simulink model "F16_Model"  (R2023b)
settings: Solver=ode4  StartTime=0.0  StopTime=inf  FixedStep=deltaTime  RelTol=1e-3
PreLoadFcn:
  | addpath(genpath(cd))
InitFcn:
  | Run_Config
undefined symbols (not defined in the file or in its folder): controlDeflections, dataBase, deltaLEF, statesFinal
libraries: simulink_extras x17, vrlib x1, sharedtransform x1
(part 1 of 2)
Description:
  | % Description   :   - Created
  | %                   - Re-arranged blocks.
  | %                   - Added reset in all integrators.
  | %                   - Created Unity Visualizer block.
  | %                   - Created G command to pitch rate
settings Model: SimulationMode=accelerator  Creator=Fatih Erol  LastModifiedBy=cyber
settings DebuggingCC: UnconnectedInputMsg=warning  UnconnectedOutputMsg=warning  UnconnectedLineMsg=warning
settings ModelReferenceCC: EnableRefExpFcnMdlSchedulingChecks=on
settings RTWCC: DLArmComputeVersion=19.05

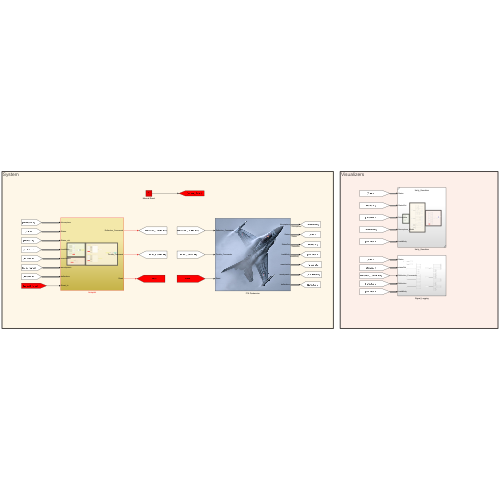
[thumbnail: Simulink's stored preview of the top-level diagram]
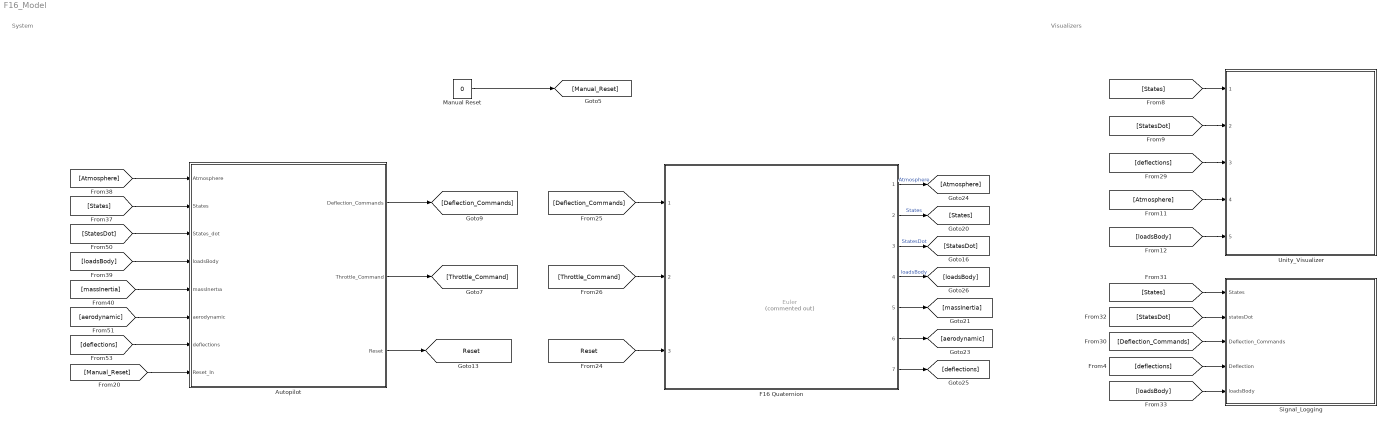
== system F16_Model ==
  note: Visualizers
  note: System
  Autopilot : Subsystem
  Euler : Subsystem  Commented=on
  F16 Quaternion : Subsystem  ReferencedSubsystem=F16_Quaternion
  Manual Reset : Constant  Value=0
      settings: OpenFcn=|
      | val = get_param(gcb,'Value')
      | 
      | switch val
      | case '1'
      | set_param(gcb,'Value','0')
      | set_param(gcb,'BackGroundColor','red')
      | otherwise
      | set_param(gcb,'Value','1')
      | set_param(gcb,'BackGroundColor','green')
      | end
  Signal_Logging : Subsystem
  Unity_Visualizer : Subsystem  ReferencedSubsystem=Unity_Visualizer
  tag scope: Reset=global
  wires:
  [States] -> Unity_Visualizer/1
  [StatesDot] -> Unity_Visualizer/2
  [deflections] -> Unity_Visualizer/3
  [Atmosphere] -> Unity_Visualizer/4
  [loadsBody] -> Unity_Visualizer/5
  [States] -> Signal_Logging/1(States)
  [Deflection_Commands] -> Signal_Logging/3(Deflection_Commands)
  [deflections] -> Signal_Logging/4(Deflection)
  [StatesDot] -> Signal_Logging/2(statesDot)
  [loadsBody] -> Signal_Logging/5(loadsBody)
  [Reset] -> F16 Quaternion/3
  [Throttle_Command] -> F16 Quaternion/2
  [Deflection_Commands] -> F16 Quaternion/1
  F16 Quaternion/7 -> [deflections]
  F16 Quaternion/6 -> [aerodynamic]
  F16 Quaternion/5 -> [massInertia]
  F16 Quaternion/4 -> [loadsBody]  "loadsBody"
  F16 Quaternion/1 -> [Atmosphere]  "Atmosphere"
  F16 Quaternion/3 -> [StatesDot]  "StatesDot"
  F16 Quaternion/2 -> [States]  "States"
  [Atmosphere] -> Autopilot/1(Atmosphere)
  [States] -> Autopilot/2(States)
  [StatesDot] -> Autopilot/3(States_dot)
  [loadsBody] -> Autopilot/4(loadsBody)
  [massInertia] -> Autopilot/5(massInertıa)
  [aerodynamic] -> Autopilot/6(aerodynamic)
  [deflections] -> Autopilot/7(deflections)
  Autopilot/2(Throttle_Command) -> [Throttle_Command]
  Autopilot/1(Deflection_Commands) -> [Deflection_Commands]
  [Manual_Reset] -> Autopilot/8(Reset_In)
  Manual Reset/1 -> [Manual_Reset]
  Autopilot/3(Reset) -> [Reset]

== system F16_Model/Autopilot ==
  note: Outputs
  note: Inputs
  note: Controllers
  Atmosphere : Inport
  States : Inport  Port=2
  States_dot : Inport  Port=3
  loadsBody : Inport  Port=4
  massInertıa : Inport  Port=5
  aerodynamic : Inport  Port=6
  deflections : Inport  Port=7
  Reset_In : Inport  Port=8
  Bus Selector : BusSelector  OutputSignals=deflectionCommands,throttleCommand
  Constant : Constant
  Controller Selector : If  IfExpression=u1 == 1  ElseIfExpressions=u1 == 2  ShowElse=off
  From19 : From  Commented=on  GotoTag=Joystick_Commands
  Joystick : Subsystem  Commented=on
  Merge : Merge
  Simulink Inputs : Subsystem
  Deflection_Commands : Outport
  Throttle_Command : Outport  Port=2
  Reset : Outport  Port=3
  wires:
  aerodynamic/1 -> [aerodynamic]
  loadsBody/1 -> [loadsBody]
  Atmosphere/1 -> [Atmosphere]
  States_dot/1 -> [StatesDot]
  deflections/1 -> [deflections]
  massInertıa/1 -> [massInertia]
  States/1 -> [States]
  [States] -> Simulink Inputs/1(States)
  [Atmosphere] -> Simulink Inputs/3(Atmosphere)
  [loadsBody] -> Simulink Inputs/4(loadsBody)
  [StatesDot] -> Simulink Inputs/2(States_dot)
  [aerodynamic] -> Simulink Inputs/5(aerodynamic)
  [massInertia] -> Simulink Inputs/6(massInertia)
  Reset_In/1 -> [Reset]
  [Reset] -> Simulink Inputs/7(Reset)
  [deflections] -> Simulink Inputs/8(deflections)
  [Manual_Controller_Commands] -> Merge/1
  [Commands] -> Bus Selector/1
  Bus Selector/1 -> Deflection_Commands/1  "<deflectionCommands>"
  Bus Selector/2 -> Throttle_Command/1  "<throttleCommand>"
  [deflections] -> Joystick/8(deflections)
  [Reset] -> Joystick/7(Reset)
  [massInertia] -> Joystick/6(massInertia)
  [aerodynamic] -> Joystick/5(aerodynamic)
  [StatesDot] -> Joystick/2(States_dot)
  [loadsBody] -> Joystick/4(loadsBody)
  [Atmosphere] -> Joystick/3(Atmosphere)
  [States] -> Joystick/1(States)
  Controller Selector/2 -> [Joystick_Controller_Active]
  Controller Selector/1 -> [Simulink_Controller_Active]
  Constant/1 -> Controller Selector/1
  [Simulink_Controller_Active] -> Simulink Inputs/Action
  [Joystick_Controller_Active] -> Joystick/Action
  [Reset] -> Reset/1
  Simulink Inputs/1(Commands) -> [Manual_Controller_Commands]
  Joystick/1(Commands) -> [Joystick_Commands]
  From19/1 -> Merge/2
  Merge/1 -> [Commands]

== system F16_Model/Euler ==
  F16 Euler Rotation : Subsystem  Commented=on
      mask Display: image('F16.PNG'); % Use "Edit Image" on toolstrip to change.
  From5 : From  Commented=on  GotoTag=Deflection_Commands
  From7 : From  Commented=on  GotoTag=Throttle_Command
  Goto : Goto  Commented=on  GotoTag=StatesDot
  Goto1 : Goto  Commented=on  GotoTag=States
  Goto11 : Goto  Commented=on  GotoTag=massInertia
  Goto12 : Goto  Commented=on  GotoTag=aerodynamic
  Goto2 : Goto  Commented=on  GotoTag=Atmosphere
  Goto3 : Goto  Commented=on  GotoTag=deflections
  Goto6 : Goto  Commented=on  GotoTag=loadsBody
  Goto8 : Goto  Commented=on  GotoTag=DCMs
  wires:
  F16 Euler Rotation/1(Atmosphere) -> Goto2/1  "Atmosphere"
  F16 Euler Rotation/4(loadsBody) -> Goto6/1  "loadsBody"
  F16 Euler Rotation/6(aerodynamic) -> Goto12/1
  F16 Euler Rotation/7(deflections) -> Goto3/1
  F16 Euler Rotation/3(StatesDot) -> Goto/1  "StatesDot"
  From5/1 -> F16 Euler Rotation/1(Deflection_Commands)
  F16 Euler Rotation/8(DCMs) -> Goto8/1
  F16 Euler Rotation/5(massInertia) -> Goto11/1
  F16 Euler Rotation/2(States) -> Goto1/1  "States"
  From7/1 -> F16 Euler Rotation/2(Throttle_Commands)

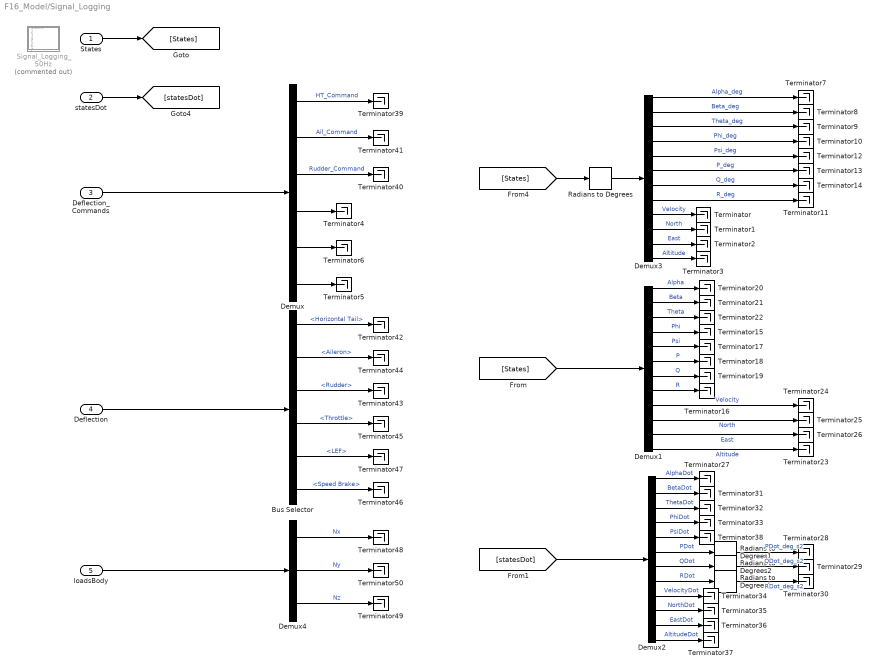
== system F16_Model/Signal_Logging ==
  States : Inport
  statesDot : Inport  Port=2
  Deflection_Commands : Inport  Port=3
  Deflection : Inport  Port=4
  loadsBody : Inport  Port=5
  Bus Selector : BusSelector  OutputSignals=Horizontal Tail,Aileron,Rudder,Throttle,LEF,Speed Brake
  Demux : Demux  Outputs=6
  Demux1 : Demux  Outputs=12
  Demux2 : Demux  Outputs=12
  Demux3 : Demux  Outputs=12
  Demux4 : Demux  Outputs=3
  Radians to Degrees{,1..3} (4 alike) : simulink_extras/Transformations/Radians to Degrees
  Signal_Logging_50Hz : Subsystem  Commented=on
  Terminator{,1..50} (51 alike) : Terminator
  wires:
  Demux3/1 -> Terminator7/1  "Alpha_deg"
  Demux3/5 -> Terminator12/1  "Psi_deg"
  Demux3/10 -> Terminator1/1  "North"
  Demux3/8 -> Terminator11/1  "R_deg"
  Demux3/9 -> Terminator/1  "Velocity"
  Demux3/4 -> Terminator10/1  "Phi_deg"
  [States] -> Radians to Degrees/1
  Demux3/7 -> Terminator14/1  "Q_deg"
  Demux3/11 -> Terminator2/1  "East"
  Demux3/6 -> Terminator13/1  "P_deg"
  Demux3/3 -> Terminator9/1  "Theta_deg"
  Radians to Degrees/1 -> Demux3/1
  Demux3/2 -> Terminator8/1  "Beta_deg"
  Demux3/12 -> Terminator3/1  "Altitude"
  States/1 -> [States]
  Deflection_Commands/1 -> Demux/1
  Demux/5 -> Terminator6/1
  Demux/2 -> Terminator41/1  "Ail_Command"
  Demux/1 -> Terminator39/1  "HT_Command"
  Demux/6 -> Terminator5/1
  Demux/4 -> Terminator4/1
  Demux/3 -> Terminator40/1  "Rudder_Command"
  [States] -> Demux1/1
  Demux1/2 -> Terminator21/1  "Beta"
  Demux1/3 -> Terminator22/1  "Theta"
  Demux1/6 -> Terminator18/1  "P"
  Demux1/7 -> Terminator19/1  "Q"
  Demux1/4 -> Terminator15/1  "Phi"
  Demux1/8 -> Terminator16/1  "R"
  Demux1/5 -> Terminator17/1  "Psi"
  Demux1/1 -> Terminator20/1  "Alpha"
  Demux1/9 -> Terminator24/1  "Velocity"
  Demux1/10 -> Terminator25/1  "North"
  Demux1/11 -> Terminator26/1  "East"
  Demux1/12 -> Terminator23/1  "Altitude"
  statesDot/1 -> [statesDot]
  Demux2/8 -> Radians to Degrees3/1  "RDot"
  Demux4/3 -> Terminator49/1  "Nz"
  [statesDot] -> Demux2/1
  Demux2/9 -> Terminator34/1  "VelocityDot"
  Demux4/2 -> Terminator50/1  "Ny"
  Demux4/1 -> Terminator48/1  "Nx"
  Demux2/5 -> Terminator38/1  "PsiDot"
  Demux2/11 -> Terminator36/1  "EastDot"
  Demux2/6 -> Radians to Degrees1/1  "PDot"
  Demux2/7 -> Radians to Degrees2/1  "QDot"
  Demux2/10 -> Terminator35/1  "NorthDot"
  Demux2/4 -> Terminator33/1  "PhiDot"
  Demux2/2 -> Terminator31/1  "BetaDot"
  Demux2/3 -> Terminator32/1  "ThetaDot"
  Demux2/1 -> Terminator27/1  "AlphaDot"
  loadsBody/1 -> Demux4/1
  Demux2/12 -> Terminator37/1  "AltitudeDot"
  Radians to Degrees1/1 -> Terminator28/1  "PDot_deg_s2"
  Radians to Degrees2/1 -> Terminator29/1  "QDot_deg_s2"
  Radians to Degrees3/1 -> Terminator30/1  "RDot_deg_s2"
  Deflection/1 -> Bus Selector/1
  Bus Selector/1 -> Terminator42/1  "<Horizontal Tail>"
  Bus Selector/2 -> Terminator44/1  "<Aileron>"
  Bus Selector/3 -> Terminator43/1  "<Rudder>"
  Bus Selector/4 -> Terminator45/1  "<Throttle>"
  Bus Selector/5 -> Terminator47/1  "<LEF>"
  Bus Selector/6 -> Terminator46/1  "<Speed Brake>"

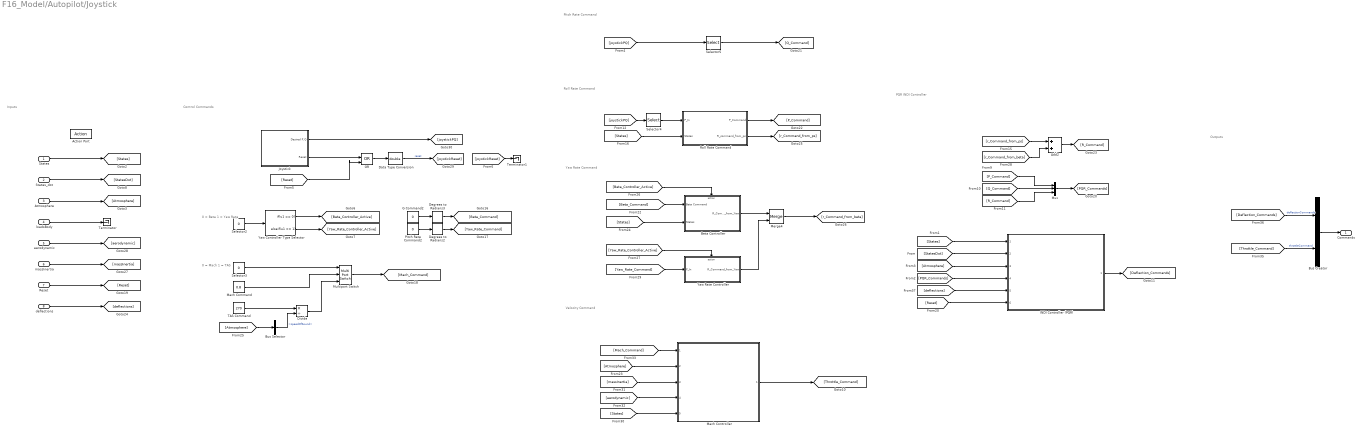
== system F16_Model/Autopilot/Joystick ==
  note: PQR INDI Controller
  note: Velocity Command
  note: Yaw Rate Command
  note: Roll Rate Command
  note: 0 = Mach
      | 1 = TAS
  note: Inputs
  note: Outputs
  note: Control Commands
  note: 0 = Beta
      | 1 = Yaw Rate
  note: Pitch Rate Command
  States : Inport
  States_dot : Inport  Port=2
  Atmosphere : Inport  Port=3
  loadsBody : Inport  Port=4
  aerodynamic : Inport  Port=5
  massInertia : Inport  Port=6
  Reset : Inport  Port=7
  deflections : Inport  Port=8
  Action Port : ActionPort  ActionPortLabel=elseif(u1 == 2)
  Add2 : Sum
  Beta Controller : Subsystem  TreatAsAtomicUnit=on
  Bus Creator : BusCreator  Inputs=2
  Bus Selector : BusSelector  OutputSignals=speedOfSound
  Data Type Conversion : DataTypeConversion  OutDataTypeStr=double  SaturateOnIntegerOverflow=off  RndMeth=Floor
  Degrees to Radians2 : simulink_extras/Transformations/Degrees to Radians
  Degrees to Radians3 : simulink_extras/Transformations/Degrees to Radians
  Divide : Product  Inputs=*/
  G Command2 : Constant  Value=0
  INDI Controller (PQR) : Subsystem  ReferencedSubsystem=INDI_Controller_PQR
  Joystick : Subsystem
  Mach Command : Constant  Value=0.8
  Mach Controller : Subsystem  ReferencedSubsystem=Mach_Controller
  Merge4 : Merge
  Multiport Switch : MultiPortSwitch  DataPortOrder=Zero-based contiguous  Inputs=2  zeroidx=on  SaturateOnIntegerOverflow=off  InputSameDT=off
  Mux : Mux  Inputs=3
  OR : Logic  Operator=OR  IconShape=distinctive  AllPortsSameDT=off  OutDataTypeStr=boolean
  Pitch Rate Command2 : Constant  Value=0
  Roll Rate Command : Subsystem
  Selector2 : Constant  Value=0
      settings: OpenFcn=|
      | val = get_param(gcb,'Value')
      | 
      | switch val
      | case '1'
      | set_param(gcb,'Value','0')
      | set_param(gcb,'BackGroundColor','red')
      | otherwise
      | set_param(gcb,'Value','1')
      | set_param(gcb,'BackGroundColor','green')
      | end
  Selector3 : Constant  Value=0
      settings: OpenFcn=|
      | val = get_param(gcb,'Value')
      | 
      | switch val
      | case '1'
      | set_param(gcb,'Value','0')
      | set_param(gcb,'BackGroundColor','red')
      | otherwise
      | set_param(gcb,'Value','1')
      | set_param(gcb,'BackGroundColor','green')
      | end
  Selector4 : Selector  InputPortWidth=2  IndexOptions=Index vector (dialog)  Indices=1  OutputSizes=1
  Selector5 : Selector  InputPortWidth=2  IndexOptions=Index vector (dialog)  Indices=2  OutputSizes=1
  TAS Command : Constant  Value=270
  Terminator : Terminator
  Terminator1 : Terminator
  Yaw Controller Type Selector : If  IfExpression=u1 == 0  ElseIfExpressions=u1 == 1  ShowElse=off
  Yaw Rate Controller : Subsystem
  Commands : Outport
  wires:
  Degrees to Radians3/1 -> [Beta_Command]
  deflections/1 -> [deflections]
  Reset/1 -> [Reset]
  INDI Controller (PQR)/1 -> [Deflection_Commands]
  Mach Controller/1 -> [Throttle_Command]
  Mach Command/1 -> Multiport Switch/2
  Divide/1 -> Multiport Switch/3
  Selector3/1 -> Multiport Switch/1
  Multiport Switch/1 -> [Mach_Command]
  TAS Command/1 -> Divide/1
  Bus Selector/1 -> Divide/2  "<speedOfSound>"
  [Atmosphere] -> Bus Selector/1
  aerodynamic/1 -> [aerodynamic]
  massInertia/1 -> [massInertia]
  [aerodynamic] -> Mach Controller/4
  [States] -> Mach Controller/5
  [Mach_Command] -> Mach Controller/1
  [massInertia] -> Mach Controller/3
  [Atmosphere] -> Mach Controller/2
  [Yaw_Rate_Controller_Active] -> Yaw Rate Controller/Action
  [Beta_Controller_Active] -> Beta Controller/Action
  [Yaw_Rate_Command] -> Yaw Rate Controller/1(P_In)
  [Beta_Command] -> Beta Controller/1(Beta Command)
  [States] -> Beta Controller/2(States)
  Beta Controller/1(R_Command_from_Yaw) -> Merge4/1
  Yaw Rate Controller/1(R_Command_from_Yaw) -> Merge4/2
  Merge4/1 -> [r_Command_from_beta]
  [States] -> Roll Rate Command/2(States)
  Add2/1 -> [R_Command]
  [r_Command_from_ps] -> Add2/1
  [r_Command_from_beta] -> Add2/2
  Selector4/1 -> Roll Rate Command/1(P_In)
  Selector5/1 -> [Q_Command]
  [R_Command] -> Mux/3
  [P_Command] -> Mux/1
  [Q_Command] -> Mux/2
  Mux/1 -> [PQR_Commands]
  Degrees to Radians2/1 -> [Yaw_Rate_Command]
  G Command2/1 -> Degrees to Radians3/1
  Pitch Rate Command2/1 -> Degrees to Radians2/1
  Yaw Controller Type Selector/2 -> [Yaw_Rate_Controller_Active]
  Yaw Controller Type Selector/1 -> [Beta_Controller_Active]
  Selector2/1 -> Yaw Controller Type Selector/1
  States_dot/1 -> [StatesDot]
  [Reset] -> INDI Controller (PQR)/6
  [PQR_Commands] -> INDI Controller (PQR)/4
  [deflections] -> INDI Controller (PQR)/5
  [States] -> INDI Controller (PQR)/1
  [StatesDot] -> INDI Controller (PQR)/2
  [Atmosphere] -> INDI Controller (PQR)/3
  States/1 -> [States]
  loadsBody/1 -> Terminator/1
  Atmosphere/1 -> [Atmosphere]
  Joystick/1(Desired P,Q) -> [joystickPQ]
  Joystick/2(Reset) -> OR/1
  [joystickPQ] -> Selector4/1
  Roll Rate Command/2(R_command_from_ps) -> [r_Command_from_ps]
  [joystickPQ] -> Selector5/1
  Roll Rate Command/1(P_Command) -> [P_Command]
  [Deflection_Commands] -> Bus Creator/1  "deflectionCommands"
  [Throttle_Command] -> Bus Creator/2  "throttleCommand"
  Bus Creator/1 -> Commands/1
  [Reset] -> OR/2
  OR/1 -> Data Type Conversion/1
  Data Type Conversion/1 -> [joystickReset]  "reset"
  [joystickReset] -> Terminator1/1

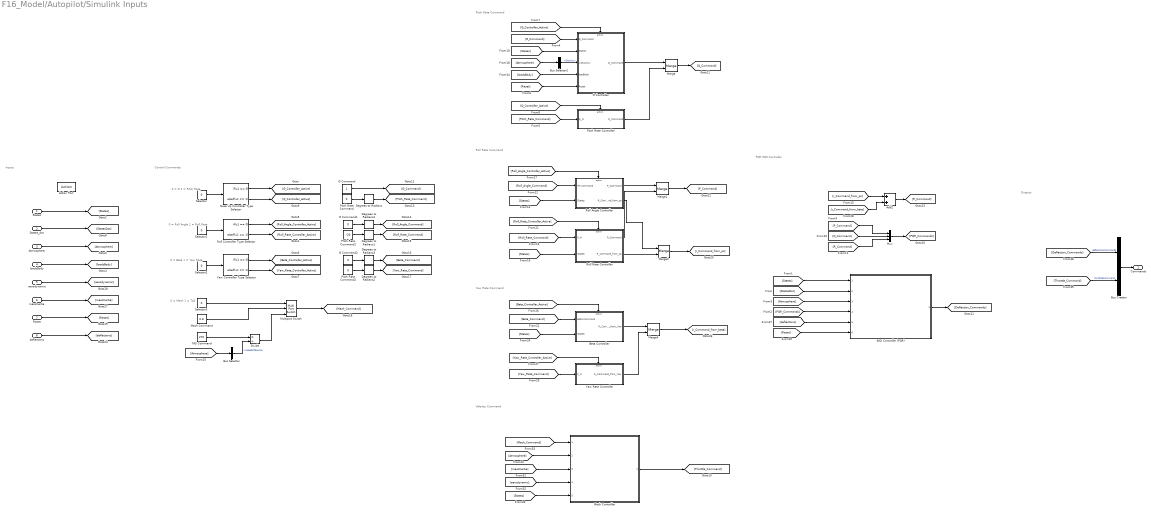
== system F16_Model/Autopilot/Simulink Inputs ==
  note: Pitch Rate Command
  note: 0 = Beta
      | 1 = Yaw Rate
  note: Control Commands
  note: Outputs
  note: Inputs
  note: 0 = G
      | 1 = Pitch Rate
  note: 0 = Roll Angle
      | 1 = Roll Rate
  note: 0 = Mach
      | 1 = TAS
  note: Roll Rate Command
  note: Yaw Rate Command
  note: Velocity Command
  note: PQR INDI Controller
  States : Inport
  States_dot : Inport  Port=2
  Atmosphere : Inport  Port=3
  loadsBody : Inport  Port=4
  aerodynamic : Inport  Port=5
  massInertia : Inport  Port=6
  Reset : Inport  Port=7
  deflections : Inport  Port=8
  Action Port : ActionPort  ActionPortLabel=if(u1 == 1)
  Add2 : Sum
  Beta Controller : Subsystem  TreatAsAtomicUnit=on
  Bus Creator : BusCreator  Inputs=2
  Bus Selector : BusSelector  OutputSignals=speedOfSound
  Bus Selector2 : BusSelector  OutputSignals=Gravity
  Degrees to Radians{,1..4} (5 alike) : simulink_extras/Transformations/Degrees to Radians
  Divide : Product  Inputs=*/
  G Command : Constant
  G Command1 : Constant  Value=0
  G Command2 : Constant  Value=0
  G Controller : Subsystem  TreatAsAtomicUnit=on
  INDI Controller (PQR) : Subsystem  ReferencedSubsystem=INDI_Controller_PQR
  Mach Command : Constant  Value=0.8
  Mach Controller : Subsystem  ReferencedSubsystem=Mach_Controller
  Merge{,1..2,4} (4 alike) : Merge
  Multiport Switch : MultiPortSwitch  DataPortOrder=Zero-based contiguous  Inputs=2  zeroidx=on  SaturateOnIntegerOverflow=off  InputSameDT=off
  Mux : Mux  Inputs=3
  Nose Up Controller Type Selector : If  IfExpression=u1 == 0  ElseIfExpressions=u1 == 1  ShowElse=off
  Pitch Rate Command : Constant  Value=0
  Pitch Rate Command1 : Constant  Value=-20
  Pitch Rate Command2 : Constant  Value=0
  Pitch Rate Controller : Subsystem  TreatAsAtomicUnit=on
  Roll Angle Controller : Subsystem  TreatAsAtomicUnit=on
  Roll Controller Type Selector : If  IfExpression=u1 == 0  ElseIfExpressions=u1 == 1  ShowElse=off
  Roll Rate Controller : Subsystem  TreatAsAtomicUnit=on
  Selector{,1..3} (4 alike) : Constant  Value=0
      settings: OpenFcn=|
      | val = get_param(gcb,'Value')
      | 
      | switch val
      | case '1'
      | set_param(gcb,'Value','0')
      | set_param(gcb,'BackGroundColor','red')
      | otherwise
      | set_param(gcb,'Value','1')
      | set_param(gcb,'BackGroundColor','green')
      | end
  TAS Command : Constant  Value=270
  Yaw Controller Type Selector : If  IfExpression=u1 == 0  ElseIfExpressions=u1 == 1  ShowElse=off
  Yaw Rate Controller : Subsystem
  Commands : Outport
  wires:
  [Atmosphere] -> Bus Selector2/1
  Atmosphere/1 -> [Atmosphere]
  loadsBody/1 -> [loadsBody]
  States/1 -> [States]
  [G_Command] -> G Controller/1(G_Command)
  [States] -> G Controller/2(States)
  Bus Selector2/1 -> G Controller/3(<Gravity>)  "<Gravity>"
  [loadsBody] -> G Controller/4(loadBody)
  [Atmosphere] -> INDI Controller (PQR)/3
  [StatesDot] -> INDI Controller (PQR)/2
  [States] -> INDI Controller (PQR)/1
  [deflections] -> INDI Controller (PQR)/5
  [PQR_Commands] -> INDI Controller (PQR)/4
  [Reset] -> INDI Controller (PQR)/6
  States_dot/1 -> [StatesDot]
  Pitch Rate Command/1 -> Degrees to Radians/1
  Selector1/1 -> Roll Controller Type Selector/1
  Selector2/1 -> Yaw Controller Type Selector/1
  Yaw Controller Type Selector/1 -> [Beta_Controller_Active]
  G Controller/1(Q_Command) -> Merge/1
  Selector/1 -> Nose Up Controller Type Selector/1
  Pitch Rate Controller/1(Q_Command) -> Merge/2
  [Pitch_Rate_Command] -> Pitch Rate Controller/1(Q_In)
  Nose Up Controller Type Selector/1 -> [G_Controller_Active]
  [G_Controller_Active] -> G Controller/Action
  Nose Up Controller Type Selector/2 -> [Q_Controller_Active]
  [Q_Controller_Active] -> Pitch Rate Controller/Action
  Roll Controller Type Selector/1 -> [Roll_Angle_Controller_Active]
  Roll Controller Type Selector/2 -> [Roll_Rate_Controller_Active]
  Yaw Controller Type Selector/2 -> [Yaw_Rate_Controller_Active]
  G Command/1 -> [G_Command]
  Degrees to Radians/1 -> [Pitch_Rate_Command]
  Degrees to Radians1/1 -> [Roll_Rate_Command]
  G Command1/1 -> Degrees to Radians4/1
  Pitch Rate Command1/1 -> Degrees to Radians1/1
  Pitch Rate Command2/1 -> Degrees to Radians2/1
  G Command2/1 -> Degrees to Radians3/1
  Degrees to Radians2/1 -> [Yaw_Rate_Command]
  Mux/1 -> [PQR_Commands]
  [Q_Command] -> Mux/2
  [P_Command] -> Mux/1
  [R_Command] -> Mux/3
  Merge/1 -> [Q_Command]
  Merge1/1 -> [P_Command]
  [Roll_Rate_Controller_Active] -> Roll Rate Controller/Action
  [Roll_Angle_Controller_Active] -> Roll Angle Controller/Action
  [Roll_Rate_Command] -> Roll Rate Controller/1(P_In)
  Roll Rate Controller/1(P_Command) -> Merge1/2
  Roll Angle Controller/1(P_Command) -> Merge1/1
  [Roll_Angle_Command] -> Roll Angle Controller/1(Phi Command)
  [States] -> Roll Angle Controller/2(States)
  [r_Command_from_beta] -> Add2/2
  [r_Command_from_ps] -> Add2/1
  Add2/1 -> [R_Command]
  [States] -> Roll Rate Controller/2(States)
  Roll Angle Controller/2(R_Command_from_ps) -> Merge2/1
  Roll Rate Controller/2(R_command_from_ps) -> Merge2/2
  Merge2/1 -> [r_Command_from_ps]
  Merge4/1 -> [r_Command_from_beta]
  Yaw Rate Controller/1(R_Command_from_Yaw) -> Merge4/2
  Beta Controller/1(R_Command_from_Yaw) -> Merge4/1
  [States] -> Beta Controller/2(States)
  [Beta_Command] -> Beta Controller/1(Beta Command)
  [Yaw_Rate_Command] -> Yaw Rate Controller/1(P_In)
  [Beta_Controller_Active] -> Beta Controller/Action
  [Yaw_Rate_Controller_Active] -> Yaw Rate Controller/Action
  [Atmosphere] -> Mach Controller/2
  [massInertia] -> Mach Controller/3
  [Mach_Command] -> Mach Controller/1
  [States] -> Mach Controller/5
  [aerodynamic] -> Mach Controller/4
  massInertia/1 -> [massInertia]
  aerodynamic/1 -> [aerodynamic]
  [Atmosphere] -> Bus Selector/1
  Bus Selector/1 -> Divide/2  "<speedOfSound>"
  TAS Command/1 -> Divide/1
  Multiport Switch/1 -> [Mach_Command]
  Selector3/1 -> Multiport Switch/1
  Divide/1 -> Multiport Switch/3
  Mach Command/1 -> Multiport Switch/2
  Mach Controller/1 -> [Throttle_Command]
  [Throttle_Command] -> Bus Creator/2  "throttleCommand"
  [Deflection_Commands] -> Bus Creator/1  "deflectionCommands"
  INDI Controller (PQR)/1 -> [Deflection_Commands]
  Reset/1 -> [Reset]
  deflections/1 -> [deflections]
  Degrees to Radians3/1 -> [Beta_Command]
  Degrees to Radians4/1 -> [Roll_Angle_Command]
  Bus Creator/1 -> Commands/1
  [Reset] -> G Controller/5(Reset)

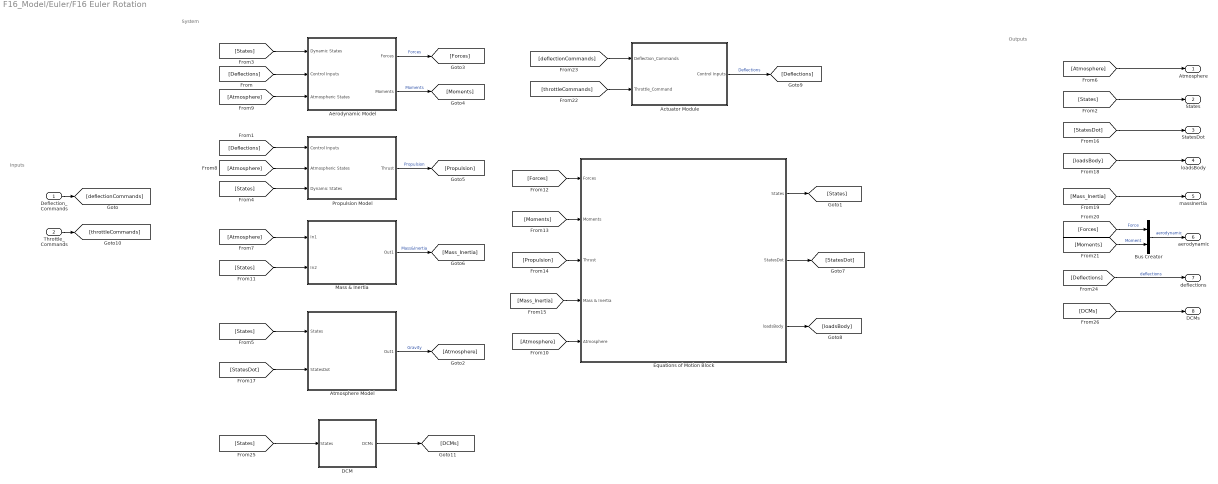
== system F16_Model/Euler/F16 Euler Rotation ==
  note: System
  note: Inputs
  note: Outputs
  Deflection_Commands : Inport
  Throttle_Commands : Inport  Port=2
  Actuator Module : Subsystem
      mask Display: image('F16_ControlSurface.png'); % Use "Edit Image" on toolstrip to change.
  Aerodynamic Model : Subsystem
      mask Display: image('F16.PNG'); % Use "Edit Image" on toolstrip to change.
  Atmosphere Model : Subsystem
      mask Display: image('f16_atm.jpg'); % Use "Edit Image" on toolstrip to change.
  Bus Creator : BusCreator  Inputs=2
  DCM : Subsystem
  Equations of Motion Block : Subsystem
      mask Display: image('F16.PNG'); % Use "Edit Image" on toolstrip to change.
  Mass & Inertia : Subsystem
      mask Display: image('F16.PNG'); % Use "Edit Image" on toolstrip to change.
  Propulsion Model : Subsystem
      mask Display: image('F16_Engine.PNG'); % Use "Edit Image" on toolstrip to change.
  Atmosphere : Outport
  States : Outport  Port=2
  StatesDot : Outport  Port=3
  loadsBody : Outport  Port=4
  massInertia : Outport  Port=5
  aerodynamic : Outport  Port=6
  deflections : Outport  Port=7
  DCMs : Outport  Port=8
  wires:
  Mass & Inertia/1(Out1) -> [Mass_Inertia]  "Mass&Inertia"
  Equations of Motion Block/1(States) -> [States]
  Aerodynamic Model/2(Moments) -> [Moments]  "Moments"
  Aerodynamic Model/1(Forces) -> [Forces]  "Forces"
  [Deflections] -> Aerodynamic Model/2(Control Inputs)
  Atmosphere Model/1(Out1) -> [Atmosphere]  "Gravity"
  Propulsion Model/1(Thrust) -> [Propulsion]  "Propulsion"
  Equations of Motion Block/2(StatesDot) -> [StatesDot]
  Deflection_Commands/1 -> [deflectionCommands]
  [Deflections] -> Propulsion Model/1(Control Inputs)
  [States] -> States/1
  [States] -> Aerodynamic Model/1(Dynamic States)
  [States] -> Propulsion Model/3(Dynamic States)
  [States] -> Atmosphere Model/1(States)
  [Atmosphere] -> Atmosphere/1
  [Atmosphere] -> Mass & Inertia/1(In1)
  [Atmosphere] -> Propulsion Model/2(Atmospheric States)
  [Atmosphere] -> Aerodynamic Model/3(Atmospheric States)
  [Atmosphere] -> Equations of Motion Block/5(Atmosphere)
  [States] -> Mass & Inertia/2(In2)
  [Forces] -> Equations of Motion Block/1(Forces)
  [Moments] -> Equations of Motion Block/2(Moments)
  [Propulsion] -> Equations of Motion Block/3(Thrust)
  [Mass_Inertia] -> Equations of Motion Block/4(Mass & Inertia)
  [StatesDot] -> StatesDot/1
  [StatesDot] -> Atmosphere Model/2(StatesDot)
  Equations of Motion Block/3(loadsBody) -> [loadsBody]
  [loadsBody] -> loadsBody/1
  [Mass_Inertia] -> massInertia/1
  [Forces] -> Bus Creator/1  "Force"
  [Moments] -> Bus Creator/2  "Moment"
  Bus Creator/1 -> aerodynamic/1  "aerodynamic"
  [throttleCommands] -> Actuator Module/2(Throttle_Command)
  Actuator Module/1(Control Inputs) -> [Deflections]  "Deflections"
  [deflectionCommands] -> Actuator Module/1(Deflection_Commands)
  Throttle_Commands/1 -> [throttleCommands]
  [Deflections] -> deflections/1  "deflections"
  [States] -> DCM/1(States)
  DCM/1(DCMs) -> [DCMs]
  [DCMs] -> DCMs/1

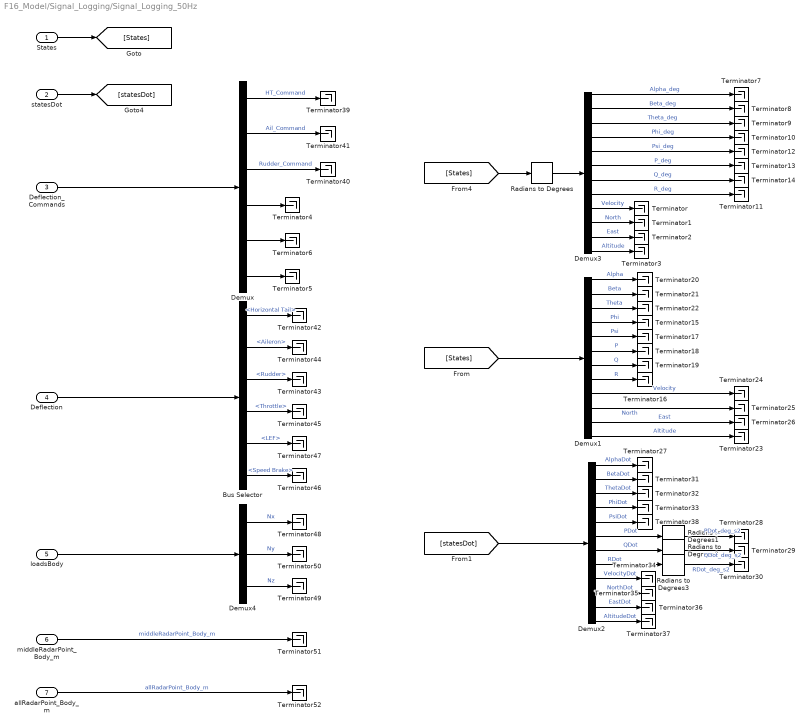
== system F16_Model/Signal_Logging/Signal_Logging_50Hz ==
  States : Inport
  statesDot : Inport  Port=2
  Deflection_Commands : Inport  Port=3
  Deflection : Inport  Port=4
  loadsBody : Inport  Port=5
  middleRadarPoint_Body_m : Inport  Port=6
  allRadarPoint_Body_m : Inport  Port=7
  Bus Selector : BusSelector  OutputSignals=Horizontal Tail,Aileron,Rudder,Throttle,LEF,Speed Brake
  Demux : Demux  Outputs=6
  Demux1 : Demux  Outputs=12
  Demux2 : Demux  Outputs=12
  Demux3 : Demux  Outputs=12
  Demux4 : Demux  Outputs=3
  Radians to Degrees{,1..3} (4 alike) : simulink_extras/Transformations/Radians to Degrees
  Terminator{,1..52} (53 alike) : Terminator
  wires:
  allRadarPoint_Body_m/1 -> Terminator52/1  "allRadarPoint_Body_m"
  middleRadarPoint_Body_m/1 -> Terminator51/1  "middleRadarPoint_Body_m"
  Bus Selector/6 -> Terminator46/1  "<Speed Brake>"
  Bus Selector/5 -> Terminator47/1  "<LEF>"
  Bus Selector/4 -> Terminator45/1  "<Throttle>"
  Bus Selector/3 -> Terminator43/1  "<Rudder>"
  Bus Selector/2 -> Terminator44/1  "<Aileron>"
  Bus Selector/1 -> Terminator42/1  "<Horizontal Tail>"
  Deflection/1 -> Bus Selector/1
  Radians to Degrees3/1 -> Terminator30/1  "RDot_deg_s2"
  Radians to Degrees2/1 -> Terminator29/1  "QDot_deg_s2"
  Radians to Degrees1/1 -> Terminator28/1  "PDot_deg_s2"
  Demux2/12 -> Terminator37/1  "AltitudeDot"
  loadsBody/1 -> Demux4/1
  Demux2/1 -> Terminator27/1  "AlphaDot"
  Demux2/3 -> Terminator32/1  "ThetaDot"
  Demux2/2 -> Terminator31/1  "BetaDot"
  Demux2/4 -> Terminator33/1  "PhiDot"
  Demux2/10 -> Terminator35/1  "NorthDot"
  Demux2/7 -> Radians to Degrees2/1  "QDot"
  Demux2/6 -> Radians to Degrees1/1  "PDot"
  Demux2/11 -> Terminator36/1  "EastDot"
  Demux2/5 -> Terminator38/1  "PsiDot"
  Demux4/1 -> Terminator48/1  "Nx"
  Demux4/2 -> Terminator50/1  "Ny"
  Demux2/9 -> Terminator34/1  "VelocityDot"
  [statesDot] -> Demux2/1
  Demux4/3 -> Terminator49/1  "Nz"
  Demux2/8 -> Radians to Degrees3/1  "RDot"
  statesDot/1 -> [statesDot]
  Demux1/12 -> Terminator23/1  "Altitude"
  Demux1/11 -> Terminator26/1  "East"
  Demux1/10 -> Terminator25/1  "North"
  Demux1/9 -> Terminator24/1  "Velocity"
  Demux1/1 -> Terminator20/1  "Alpha"
  Demux1/5 -> Terminator17/1  "Psi"
  Demux1/8 -> Terminator16/1  "R"
  Demux1/4 -> Terminator15/1  "Phi"
  Demux1/7 -> Terminator19/1  "Q"
  Demux1/6 -> Terminator18/1  "P"
  Demux1/3 -> Terminator22/1  "Theta"
  Demux1/2 -> Terminator21/1  "Beta"
  [States] -> Demux1/1
  Demux/3 -> Terminator40/1  "Rudder_Command"
  Demux/4 -> Terminator4/1
  Demux/6 -> Terminator5/1
  Demux/1 -> Terminator39/1  "HT_Command"
  Demux/2 -> Terminator41/1  "Ail_Command"
  Demux/5 -> Terminator6/1
  Deflection_Commands/1 -> Demux/1
  States/1 -> [States]
  Demux3/12 -> Terminator3/1  "Altitude"
  Demux3/2 -> Terminator8/1  "Beta_deg"
  Radians to Degrees/1 -> Demux3/1
  Demux3/3 -> Terminator9/1  "Theta_deg"
  Demux3/6 -> Terminator13/1  "P_deg"
  Demux3/11 -> Terminator2/1  "East"
  Demux3/7 -> Terminator14/1  "Q_deg"
  [States] -> Radians to Degrees/1
  Demux3/4 -> Terminator10/1  "Phi_deg"
  Demux3/9 -> Terminator/1  "Velocity"
  Demux3/8 -> Terminator11/1  "R_deg"
  Demux3/10 -> Terminator1/1  "North"
  Demux3/5 -> Terminator12/1  "Psi_deg"
  Demux3/1 -> Terminator7/1  "Alpha_deg"

== system F16_Model/Autopilot/Joystick/Beta Controller ==
  Beta Command : Inport
  States : Inport  Port=2
  Action Port : ActionPort  ActionPortLabel=if(u1 == 0)
  Beta Controller : Subsystem  ReferencedSubsystem=Beta_Controller
  R_Command_from_Yaw : Outport
  wires:
  States/1 -> [States]
  [r_Command_from_beta] -> R_Command_from_Yaw/1
  Beta Command/1 -> [Beta_command]
  [Beta_command] -> Beta Controller/1
  [States] -> Beta Controller/2
  Beta Controller/1 -> [r_Command_from_beta]

== system F16_Model/Autopilot/Joystick/Joystick ==
  1-D Lookup Table : Lookup_n-D  NumberOfTableDimensions=1  BreakpointsForDimension1=[-1,1]  Table=[-40,40]  InternalRulePriority=Speed  RndMeth=Simplest
  1-D Lookup Table1 : Lookup_n-D  NumberOfTableDimensions=1  BreakpointsForDimension1=[-1,1]  Table=[-180,180]  InternalRulePriority=Speed  RndMeth=Simplest
  Data Type Conversion2 : DataTypeConversion  SaturateOnIntegerOverflow=off  RndMeth=Floor
  Data Type Conversion3 : DataTypeConversion  SaturateOnIntegerOverflow=off  RndMeth=Floor
  Degrees to Radians2 : simulink_extras/Transformations/Degrees to Radians
  Degrees to Radians3 : simulink_extras/Transformations/Degrees to Radians
  Demux : Demux  Outputs=2
  Joystick Input : vrlib/Joystick Input  joyid=1  adjustports=on  forcefeed=off
  Mux : Mux  Inputs=2
  Selector : Selector  IndexOptions=Index vector (dialog)  Indices=4  OutputSizes=1
  Terminator : Terminator
  Desired P,Q : Outport
  Reset : Outport  Port=2
  wires:
  Data Type Conversion2/1 -> Reset/1  "Reset"
  Demux/2 -> 1-D Lookup Table/1
  Degrees to Radians3/1 -> Mux/2
  Data Type Conversion3/1 -> Data Type Conversion2/1
  Demux/1 -> 1-D Lookup Table1/1
  Joystick Input/1 -> Demux/1
  Degrees to Radians2/1 -> Mux/1
  1-D Lookup Table1/1 -> Degrees to Radians2/1  "Roll Rate Demand"
  Mux/1 -> Desired P,Q/1  "Desired P,Q"
  Selector/1 -> Data Type Conversion3/1
  1-D Lookup Table/1 -> Degrees to Radians3/1
  Joystick Input/2 -> Selector/1
  ? -> Terminator/1

== system F16_Model/Autopilot/Joystick/Roll Rate Command ==
  P_In : Inport
  States : Inport  Port=2
  Bus Selector : BusSelector  OutputSignals=Alpha
  Cos : Trigonometry  Operator=cos
  Cos1 : Trigonometry  Operator=tan
  Gain : Gain
  Product : Product
  Product1 : Product
  P_Command : Outport
  R_command_from_ps : Outport  Port=2
  wires:
  States/1 -> Bus Selector/1
  Gain/1 -> P_Command/1
  Cos1/1 -> Product1/1
  P_In/1 -> Gain/1, Product/2
  Product1/1 -> R_command_from_ps/1
  Product/1 -> Product1/2
  Bus Selector/1 -> Cos/1, Cos1/1  "<Alpha>"
  Cos/1 -> Product/1

== system F16_Model/Autopilot/Joystick/Yaw Rate Controller ==
  P_In : Inport
  Action Port : ActionPort  ActionPortLabel=elseif(u1 == 1)
  R_Command_from_Yaw : Outport
  wires:
  P_In/1 -> R_Command_from_Yaw/1

== system F16_Model/Autopilot/Simulink Inputs/Beta Controller ==
  Beta Command : Inport
  States : Inport  Port=2
  Action Port : ActionPort  ActionPortLabel=if(u1 == 0)
  Beta Controller : Subsystem  ReferencedSubsystem=Beta_Controller
  R_Command_from_Yaw : Outport
  wires:
  States/1 -> [States]
  [r_Command_from_beta] -> R_Command_from_Yaw/1
  Beta Command/1 -> [Beta_command]
  [Beta_command] -> Beta Controller/1
  [States] -> Beta Controller/2
  Beta Controller/1 -> [r_Command_from_beta]

== system F16_Model/Autopilot/Simulink Inputs/G Controller ==
  G_Command : Inport
  States : Inport  Port=2
  <Gravity> : Inport  Port=3
  loadBody : Inport  Port=4
  Reset : Inport  Port=5
  Action Port : ActionPort  ActionPortLabel=if(u1 == 0)
  G Command to PQR Command : Subsystem  ReferencedSubsystem=G_Command_to_PQR_Command
  Q_Command : Outport
  wires:
  G Command to PQR Command/1 -> Q_Command/1  "Q_Command"
  loadBody/1 -> G Command to PQR Command/4
  <Gravity>/1 -> G Command to PQR Command/3
  G_Command/1 -> G Command to PQR Command/1
  States/1 -> G Command to PQR Command/2
  Reset/1 -> G Command to PQR Command/5

== system F16_Model/Autopilot/Simulink Inputs/Pitch Rate Controller ==
  Q_In : Inport
  Action Port : ActionPort  ActionPortLabel=elseif(u1 == 1)
  Q_Command : Outport
  wires:
  Q_In/1 -> Q_Command/1

== system F16_Model/Autopilot/Simulink Inputs/Roll Angle Controller ==
  Phi Command : Inport
  States : Inport  Port=2
  Action Port : ActionPort  ActionPortLabel=if(u1 == 0)
  "Roll Angle Hold Auto Pilot " : Subsystem  ReferencedSubsystem=Roll_Angle_Hold_Auto_Pilot
  P_Command : Outport
  R_Command_from_ps : Outport  Port=2
  wires:
  "Roll Angle Hold Auto Pilot "/2 -> [R_Command_from_ps]
  "Roll Angle Hold Auto Pilot "/1 -> [P_Command]
  [phi_Command] -> "Roll Angle Hold Auto Pilot "/2
  [States] -> "Roll Angle Hold Auto Pilot "/1
  Phi Command/1 -> [phi_Command]
  [P_Command] -> P_Command/1
  [R_Command_from_ps] -> R_Command_from_ps/1
  States/1 -> [States]

== system F16_Model/Autopilot/Simulink Inputs/Roll Rate Controller ==
  P_In : Inport
  States : Inport  Port=2
  Action Port : ActionPort  ActionPortLabel=elseif(u1 == 1)
  Roll Rate Command : Subsystem
  P_Command : Outport
  R_command_from_ps : Outport  Port=2
  wires:
  P_In/1 -> Roll Rate Command/1(P_In)
  States/1 -> Roll Rate Command/2(States)
  Roll Rate Command/1(P_Command) -> P_Command/1
  Roll Rate Command/2(R_command_from_ps) -> R_command_from_ps/1

== system F16_Model/Autopilot/Simulink Inputs/Yaw Rate Controller ==
  P_In : Inport
  Action Port : ActionPort  ActionPortLabel=elseif(u1 == 1)
  R_Command_from_Yaw : Outport
  wires:
  P_In/1 -> R_Command_from_Yaw/1

== system F16_Model/Euler/F16 Euler Rotation/Actuator Module ==
  Deflection_Commands : Inport
  Throttle_Command : Inport  Port=2
  Bus Creator : BusCreator  Inputs=6
  Demux : Demux  Outputs=6
  First Order Aileron Actuator : Subsystem
  First Order HT Actuator : Subsystem
  First Order Rudder Actuator : Subsystem
  First Order Throttle Actuator : Subsystem
  Leading Edge Flap : Constant  Value=deltaLEF
  Speed Brake : Constant  Value=0
  Terminator : Terminator
  Terminator1 : Terminator
  Terminator2 : Terminator
  Control Inputs : Outport
  wires:
  Bus Creator/1 -> Control Inputs/1
  First Order Throttle Actuator/1(Output) -> Bus Creator/4  "Throttle"
  Speed Brake/1 -> Bus Creator/6  "Speed Brake"
  Demux/1 -> [HorizontalTail]
  Demux/2 -> [Aileron]
  Demux/3 -> [Rudder]
  Demux/4 -> Terminator/1
  Demux/5 -> Terminator2/1
  Demux/6 -> Terminator1/1
  Deflection_Commands/1 -> Demux/1
  Leading Edge Flap/1 -> Bus Creator/5  "LEF"
  [HorizontalTail] -> First Order HT Actuator/1(Deflection)  "Horizontal Tail Command"
  [Aileron] -> First Order Aileron Actuator/1(Deflection)  "Aileron Command"
  [Rudder] -> First Order Rudder Actuator/1(Deflection)  "Rudder Command"
  First Order HT Actuator/1(Output) -> Bus Creator/1  "Horizontal Tail"
  First Order Aileron Actuator/1(Output) -> Bus Creator/2  "Aileron"
  First Order Rudder Actuator/1(Output) -> Bus Creator/3  "Rudder"
  Throttle_Command/1 -> [Throttle_Command]
  [Throttle_Command] -> First Order Throttle Actuator/1(Deflection)  "Throttle Command"

== system F16_Model/Euler/F16 Euler Rotation/Aerodynamic Model ==
  Dynamic States : Inport
  Control Inputs : Inport  Port=2
  Atmospheric States : Inport  Port=3
  Bus Creator : BusCreator  Inputs=2
  Bus Selector : BusSelector  OutputSignals=Dynamic Pressure
  Constant : Constant  Value=dataBase.Sw
  Demux1 : Demux  Outputs=3
  Force Coeffs : Subsystem
  Gain : Gain  Gain=dataBase.MAC*dataBase.Sw
  Gain1 : Gain  Gain=dataBase.b*dataBase.Sw
  Gain2 : Gain  Gain=dataBase.b*dataBase.Sw
  Moment Coeffs : Subsystem
  Mux : Mux  Inputs=3
  Mux1 : Mux  Inputs=3
  Mux2 : Mux  Inputs=3
  Product : Product  Inputs=3
  Product1 : Product
  Product2 : Product
  Product3 : Product
  Forces : Outport
  Moments : Outport  Port=2
  wires:
  Force Coeffs/3(" CZ") -> Bus Creator/2, Mux/3  "CZ"
  Force Coeffs/2(" CY") -> Bus Creator/1, Mux/2  "CY"
  Force Coeffs/1(" CX") -> Mux/1
  Mux/1 -> Product/2
  Moment Coeffs/1(" Cm") -> Mux1/1
  Mux1/1 -> Demux1/1
  Moment Coeffs/3(" Cn") -> Mux1/3
  Moment Coeffs/2(" Cl") -> Mux1/2
  Bus Creator/1 -> Moment Coeffs/1(Force Effects on Moments)
  Dynamic States/1 -> Moment Coeffs/2(Dynamic States), Force Coeffs/1(Dynamic States)
  Control Inputs/1 -> Moment Coeffs/3(Control Inputs), Force Coeffs/2(Control Inputs)
  Atmospheric States/1 -> Bus Selector/1
  Bus Selector/1 -> [DynamicPressure]  "<Dynamic Pressure>"
  [DynamicPressure] -> Product/1
  Constant/1 -> Product/3
  Product/1 -> Forces/1
  Demux1/1 -> Gain/1
  Gain/1 -> Product1/2
  [DynamicPressure] -> Product2/1, Product3/1, Product1/1
  Demux1/2 -> Gain1/1
  Demux1/3 -> Gain2/1
  Gain1/1 -> Product2/2
  Gain2/1 -> Product3/2
  Product3/1 -> Mux2/3
  Product2/1 -> Mux2/2
  Product1/1 -> Mux2/1
  Mux2/1 -> Moments/1

== system F16_Model/Euler/F16 Euler Rotation/Atmosphere Model ==
  States : Inport
  StatesDot : Inport  Port=2
  Add : Sum
  Atan2 : Trigonometry  Operator=atan2
  Bus Creator : BusCreator  Inputs=7
  Bus Selector : BusSelector  OutputSignals=Altitude,Velocity
  Bus Selector1 : BusSelector  OutputSignals=AltitudeDot,NorthDot,EastDot
  MATLAB Function : MATLAB Function  TreatAsAtomicUnit=on
  Sqrt : Sqrt
  Square : Math  Operator=square
  Square1 : Math  Operator=square
  Out1 : Outport
  wires:
  States/1 -> Bus Selector/1
  MATLAB Function/2(T) -> Bus Creator/2  "Temperature"
  MATLAB Function/3(P) -> Bus Creator/3  "Pressure"
  MATLAB Function/4(rho) -> Bus Creator/4  "Density"
  MATLAB Function/5(Qdyn) -> Bus Creator/5  "Dynamic Pressure"
  MATLAB Function/6(M) -> Bus Creator/6  "Mach"
  MATLAB Function/1(g) -> Bus Creator/1  "Gravity"
  Bus Creator/1 -> Out1/1
  Bus Selector/1 -> MATLAB Function/1(h)  "<Altitude>"
  Bus Selector/2 -> MATLAB Function/2(V)  "<Velocity>"
  StatesDot/1 -> Bus Selector1/1
  Bus Selector1/2 -> Square/1  "<NorthDot>"
  Bus Selector1/3 -> Square1/1  "<EastDot>"
  Bus Selector1/1 -> Atan2/1  "<AltitudeDot>"
  Square/1 -> Add/1
  Square1/1 -> Add/2
  Add/1 -> Sqrt/1
  Sqrt/1 -> Atan2/2
  Atan2/1 -> Bus Creator/7  "gamma_rad"

== system F16_Model/Euler/F16 Euler Rotation/DCM ==
  note: psi,theta,phi be means earth to body
  States : Inport
  Bus Creator : BusCreator  Inputs=1
  Bus Selector : BusSelector  OutputSignals=Phi,Theta,Psi
  Mux : Mux  Inputs=3
  Rotation Angles to Direction Cosine Matrix : sharedtransform/Rotation Angles to Direction Cosine Matrix  rotationOrder=ZYX  aMode=aMode
  DCMs : Outport
  wires:
  Mux/1 -> Rotation Angles to Direction Cosine Matrix/1
  States/1 -> Bus Selector/1
  Bus Selector/1 -> [phi]  "<Phi>"
  Bus Selector/2 -> [theta]  "<Theta>"
  Bus Selector/3 -> [psi]  "<Psi>"
  [theta] -> Mux/2
  [phi] -> Mux/3
  [psi] -> Mux/1
  Rotation Angles to Direction Cosine Matrix/1 -> Bus Creator/1  "DCMbe"
  Bus Creator/1 -> DCMs/1

== system F16_Model/Euler/F16 Euler Rotation/Equations of Motion Block ==
  note: Outputs
  note: System
  note: Inputs
  Forces : Inport
  Moments : Inport  Port=2
  Thrust : Inport  Port=3
  Mass & Inertia : Inport  Port=4
  Atmosphere : Inport  Port=5
  Bus Creator : BusCreator  Inputs=3
  Bus Creator1 : BusCreator  Inputs=12
  Bus Creator2 : BusCreator  Inputs=12
  Bus Selector : BusSelector  OutputSignals=Gravity
  Demux : Demux  Outputs=12
  Demux1 : Demux  Outputs=12
  Demux2 : Demux  Outputs=3
  F16 EoM : MATLAB Function  TreatAsAtomicUnit=on
  Integrator : Integrator  ExternalReset=either  InitialCondition=statesFinal  ContinuousStateAttributes='states'
  States : Outport
  StatesDot : Outport  Port=2
  loadsBody : Outport  Port=3
  wires:
  F16 EoM/1(xDot) -> Integrator/1, [StatesDot]
  Thrust/1 -> F16 EoM/3(Thrust)
  Integrator/1 -> [States]  "State Propagation"
  Bus Creator1/1 -> States/1
  Demux/1 -> Bus Creator1/1  "Alpha"
  Demux/2 -> Bus Creator1/2  "Beta"
  Demux/3 -> Bus Creator1/3  "Theta"
  Demux/4 -> Bus Creator1/4  "Phi"
  Demux/5 -> Bus Creator1/5  "Psi"
  Demux/6 -> Bus Creator1/6  "P"
  Demux/12 -> Bus Creator1/12  "Altitude"
  Demux/11 -> Bus Creator1/11  "East"
  Demux/10 -> Bus Creator1/10  "North"
  Demux/9 -> Bus Creator1/9  "Velocity"
  Demux/8 -> Bus Creator1/8  "R"
  Demux/7 -> Bus Creator1/7  "Q"
  Forces/1 -> F16 EoM/1(Forces)
  Moments/1 -> F16 EoM/2(Moments)
  Mass & Inertia/1 -> F16 EoM/4(Mass_Inertia)
  Atmosphere/1 -> Bus Selector/1
  Bus Creator2/1 -> StatesDot/1
  Demux1/1 -> Bus Creator2/1  "AlphaDot"
  Demux1/2 -> Bus Creator2/2  "BetaDot"
  Demux1/3 -> Bus Creator2/3  "ThetaDot"
  Demux1/4 -> Bus Creator2/4  "PhiDot"
  Demux1/5 -> Bus Creator2/5  "PsiDot"
  Demux1/12 -> Bus Creator2/12  "AltitudeDot"
  Demux1/11 -> Bus Creator2/11  "EastDot"
  Demux1/10 -> Bus Creator2/10  "NorthDot"
  Demux1/9 -> Bus Creator2/9  "VelocityDot"
  F16 EoM/2(loadsBody) -> [loadsBody]
  [States] -> Demux/1
  [StatesDot] -> Demux1/1
  Demux1/6 -> Bus Creator2/6  "PDot"
  Demux1/7 -> Bus Creator2/7  "QDot"
  Demux1/8 -> Bus Creator2/8  "RDot"
  [States] -> F16 EoM/6(states)
  Bus Selector/1 -> F16 EoM/5(Gravity)  "<Gravity>"
  [loadsBody] -> Demux2/1
  Demux2/1 -> Bus Creator/1  "Nx"
  Demux2/2 -> Bus Creator/2  "Ny"
  Demux2/3 -> Bus Creator/3  "Nz"
  Bus Creator/1 -> loadsBody/1
  [Reset] -> Integrator/2

== system F16_Model/Euler/F16 Euler Rotation/Mass & Inertia ==
  In1 : Inport
  In2 : Inport  Port=2
  Bus Creator : BusCreator  Inputs=6
  Bus Selector : BusSelector  OutputSignals=Gravity
  Bus Selector1 : BusSelector  OutputSignals=Theta,Phi
  MATLAB Function : MATLAB Function  TreatAsAtomicUnit=on
  Out1 : Outport
  wires:
  In1/1 -> Bus Selector/1
  Bus Selector/1 -> MATLAB Function/1(g)  "<Gravity>"
  In2/1 -> Bus Selector1/1
  Bus Selector1/1 -> MATLAB Function/2(theta)  "<Theta>"
  Bus Selector1/2 -> MATLAB Function/3(phi)  "<Phi>"
  MATLAB Function/1(Mass) -> Bus Creator/1
  MATLAB Function/2(Ixx) -> Bus Creator/2
  MATLAB Function/3(Iyy) -> Bus Creator/3
  MATLAB Function/4(Izz) -> Bus Creator/4
  MATLAB Function/5(Ixz) -> Bus Creator/5
  MATLAB Function/6(Fg_body) -> Bus Creator/6
  Bus Creator/1 -> Out1/1

== system F16_Model/Euler/F16 Euler Rotation/Propulsion Model ==
  Control Inputs : Inport
  Atmospheric States : Inport  Port=2
  Dynamic States : Inport  Port=3
  Bus Creator : BusCreator  Inputs=2
  Bus Selector3 : BusSelector  OutputSignals=Throttle
  Bus Selector4 : BusSelector  OutputSignals=Mach
  Bus Selector5 : BusSelector  OutputSignals=Altitude,Q,R
  Gain1 : Gain  Gain=4.4882
  Gain2 : Gain  Gain=4.4882
  Gain3 : Gain  Gain=4.4882
  Idle : Lookup_n-D  BreakpointsForDimension1=dataBase.Engine.f16_EngineData.BP.idle.mach  BreakpointsForDimension2=dataBase.Engine.f16_EngineData.BP.idle.alt_ft  Table=dataBase.Engine.f16_EngineData.data.Thrust_lbs.idle  ExtrapMethod=Clip  InternalRulePriority=Speed  RndMeth=Simplest
      settings: InputPortMap=u0,u1
  MATLAB Function : MATLAB Function  TreatAsAtomicUnit=on
  MATLAB Function1 : MATLAB Function  TreatAsAtomicUnit=on
  Maximum : Lookup_n-D  BreakpointsForDimension1=dataBase.Engine.f16_EngineData.BP.max.mach  BreakpointsForDimension2=dataBase.Engine.f16_EngineData.BP.max.alt_ft  Table=dataBase.Engine.f16_EngineData.data.Thrust_lbs.max  ExtrapMethod=Clip  InternalRulePriority=Speed  RndMeth=Simplest
      settings: InputPortMap=u0,u1
  Military : Lookup_n-D  BreakpointsForDimension1=dataBase.Engine.f16_EngineData.BP.mil.mach  BreakpointsForDimension2=dataBase.Engine.f16_EngineData.BP.mil.alt_ft  Table=dataBase.Engine.f16_EngineData.data.Thrust_lbs.mil  ExtrapMethod=Clip  InternalRulePriority=Speed  RndMeth=Simplest
      settings: InputPortMap=u0,u1
  m2ft : Gain  Gain=1/0.3048
  Thrust : Outport
  wires:
  [Tidle] -> MATLAB Function1/1(Tidle)
  [Tmil] -> MATLAB Function1/2(Tmil)
  Gain3/1 -> [Tmax]
  Idle/1 -> Gain1/1
  Gain1/1 -> [Tidle]
  Maximum/1 -> Gain3/1
  Military/1 -> Gain2/1
  [Tmax] -> MATLAB Function1/3(Tmax)
  m2ft/1 -> Maximum/2, Military/2, Idle/2
  Gain2/1 -> [Tmil]
  Control Inputs/1 -> Bus Selector3/1
  Bus Selector3/1 -> MATLAB Function1/4(Throttle)  "<Throttle>"
  Bus Selector4/1 -> Maximum/1, Military/1, Idle/1  "<Mach>"
  Bus Selector5/1 -> m2ft/1  "<Altitude>"
  Dynamic States/1 -> Bus Selector5/1
  Atmospheric States/1 -> Bus Selector4/1
  Bus Selector5/2 -> [Q]  "<Q>"
  Bus Selector5/3 -> [R]  "<R>"
  [Q] -> MATLAB Function/1(Q)
  [R] -> MATLAB Function/2(R)
  Bus Creator/1 -> Thrust/1
  MATLAB Function1/1(Thrust) -> Bus Creator/1
  MATLAB Function/1(T_moment) -> Bus Creator/2

== system F16_Model/Autopilot/Simulink Inputs/Roll Rate Controller/Roll Rate Command ==
  P_In : Inport
  States : Inport  Port=2
  Bus Selector : BusSelector  OutputSignals=Alpha
  Cos : Trigonometry  Operator=cos
  Cos1 : Trigonometry  Operator=tan
  Gain : Gain
  Product : Product
  Product1 : Product
  P_Command : Outport
  R_command_from_ps : Outport  Port=2
  wires:
  Cos/1 -> Product/1
  Bus Selector/1 -> Cos1/1, Cos/1  "<Alpha>"
  Product/1 -> Product1/2
  Product1/1 -> R_command_from_ps/1
  P_In/1 -> Product/2, Gain/1
  Cos1/1 -> Product1/1
  Gain/1 -> P_Command/1
  States/1 -> Bus Selector/1

== system F16_Model/Euler/F16 Euler Rotation/Actuator Module/First Order Aileron Actuator ==
  Deflection : Inport
  Gain : Gain  Gain=1/0.0495
  Integrator : Integrator  ExternalReset=either  InitialCondition=controlDeflections(2)
  Saturation : Saturate  UpperLimit=20  LowerLimit=-20
  Saturation1 : Saturate  UpperLimit=60  LowerLimit=-60
  Sum1 : Sum  Inputs=|+-
  Output : Outport
  wires:
  Saturation1/1 -> Integrator/1
  Gain/1 -> Saturation1/1
  Sum1/1 -> Gain/1
  Deflection/1 -> Sum1/1
  Integrator/1 -> Saturation/1
  Saturation/1 -> Output/1, Sum1/2
  [Reset] -> Integrator/2

== system F16_Model/Euler/F16 Euler Rotation/Actuator Module/First Order HT Actuator ==
  Deflection : Inport
  Gain : Gain  Gain=1/0.0495
  Integrator : Integrator  ExternalReset=either  InitialCondition=controlDeflections(1)
  Saturation : Saturate  UpperLimit=25  LowerLimit=-25
  Saturation1 : Saturate  UpperLimit=60  LowerLimit=-60
  Sum1 : Sum  Inputs=|+-
  Output : Outport
  wires:
  Sum1/1 -> Gain/1
  Gain/1 -> Saturation1/1
  Integrator/1 -> Saturation/1
  Saturation1/1 -> Integrator/1
  Deflection/1 -> Sum1/1
  Saturation/1 -> Output/1, Sum1/2
  [Reset] -> Integrator/2

== system F16_Model/Euler/F16 Euler Rotation/Actuator Module/First Order Rudder Actuator ==
  Deflection : Inport
  Gain : Gain  Gain=1/0.0495
  Integrator : Integrator  ExternalReset=either  InitialCondition=controlDeflections(3)
  Saturation : Saturate  UpperLimit=30  LowerLimit=-30
  Saturation1 : Saturate  UpperLimit=120  LowerLimit=-120
  Sum1 : Sum  Inputs=|+-
  Output : Outport
  wires:
  Sum1/1 -> Gain/1
  Gain/1 -> Saturation1/1
  Saturation/1 -> Output/1, Sum1/2
  Saturation1/1 -> Integrator/1
  Deflection/1 -> Sum1/1
  Integrator/1 -> Saturation/1
  [Reset] -> Integrator/2

== system F16_Model/Euler/F16 Euler Rotation/Actuator Module/First Order Throttle Actuator ==
  Deflection : Inport
  Gain : Gain  Gain=1/0.0495
  Integrator : Integrator  ExternalReset=either  InitialCondition=controlDeflections(4)
  Saturation : Saturate  UpperLimit=100  LowerLimit=0
  Saturation1 : Saturate  UpperLimit=30  LowerLimit=-30
  Sum1 : Sum  Inputs=|+-
  Output : Outport
  wires:
  [Reset] -> Integrator/2
  Integrator/1 -> Saturation/1
  Deflection/1 -> Sum1/1
  Saturation1/1 -> Integrator/1
  Saturation/1 -> Sum1/2, Output/1
  Gain/1 -> Saturation1/1
  Sum1/1 -> Gain/1

== system F16_Model/Euler/F16 Euler Rotation/Aerodynamic Model/Force Coeffs ==
  Dynamic States : Inport
  Control Inputs : Inport  Port=2
  Bus Creator : BusCreator  Inputs=7
  Bus Creator1 : BusCreator  Inputs=7
  Bus Creator2 : BusCreator  Inputs=8
  Bus Selector : BusSelector  OutputSignals=Alpha,Beta,P,Q,R,Velocity
  Bus Selector1 : BusSelector  OutputSignals=Horizontal Tail,Aileron,Rudder,LEF,Speed Brake
  Display : Display
  Display1 : Display
  Display2 : Display
  Gain : Gain  Gain=180/pi
  Gain1 : Gain  Gain=180/pi
  X-Axis Force : Subsystem
  Y-Axis Force : Subsystem
  Z-Axis Force : Subsystem
  " CX" : Outport  VectorParamsAs1DForOutWhenUnconnected=off
  " CY" : Outport  Port=2  VectorParamsAs1DForOutWhenUnconnected=off
  " CZ" : Outport  Port=3  VectorParamsAs1DForOutWhenUnconnected=off
  wires:
  Dynamic States/1 -> Bus Selector/1
  Bus Creator/1 -> X-Axis Force/1(States)
  X-Axis Force/1(CX) -> Display/1, " CX"/1
  Y-Axis Force/1(CY) -> Display1/1, " CY"/1
  Z-Axis Force/1(CZ) -> Display2/1, " CZ"/1
  [Alpha_deg] -> Bus Creator/1  "Alpha"
  [Beta_deg] -> Bus Creator/2  "Beta"
  [LeadingEdgeFlap] -> Bus Creator/3
  [Q] -> Bus Creator/4
  [SpeedBrake] -> Bus Creator/5
  [HorizontalTail] -> Bus Creator/6
  [Velocity] -> Bus Creator/7
  [Velocity] -> Bus Creator1/7
  [HorizontalTail] -> Bus Creator1/6
  [SpeedBrake] -> Bus Creator1/5
  [Q] -> Bus Creator1/4
  [LeadingEdgeFlap] -> Bus Creator1/3
  Bus Creator1/1 -> Z-Axis Force/1(States)
  [LeadingEdgeFlap] -> Bus Creator2/3
  [R] -> Bus Creator2/4
  [Rudder] -> Bus Creator2/6
  [Velocity] -> Bus Creator2/7
  Bus Creator2/1 -> Y-Axis Force/1(States)
  [Aileron] -> Bus Creator2/8
  [P] -> Bus Creator2/5
  Bus Selector/1 -> [Alpha]  "<Alpha>"
  Bus Selector/2 -> [Beta]  "<Beta>"
  Bus Selector/3 -> [P]  "<P>"
  Bus Selector/4 -> [Q]  "<Q>"
  Bus Selector/5 -> [R]  "<R>"
  Bus Selector/6 -> [Velocity]  "<Velocity>"
  Control Inputs/1 -> Bus Selector1/1
  Bus Selector1/1 -> [HorizontalTail]  "<Horizontal Tail>"
  Bus Selector1/2 -> [Aileron]  "<Aileron>"
  Bus Selector1/3 -> [Rudder]  "<Rudder>"
  Bus Selector1/4 -> [LeadingEdgeFlap]  "<LEF>"
  Bus Selector1/5 -> [SpeedBrake]  "<Speed Brake>"
  [Alpha] -> Gain/1
  Gain/1 -> [Alpha_deg]
  [Beta] -> Gain1/1
  Gain1/1 -> [Beta_deg]
  [Alpha_deg] -> Bus Creator2/1  "Alpha"
  [Beta_deg] -> Bus Creator2/2  "Beta"
  [Alpha_deg] -> Bus Creator1/1  "Alpha"
  [Beta_deg] -> Bus Creator1/2  "Beta"
